simulink model "stateflow_incrementsaction"  (R2015b)
settings: Solver=VariableStepAuto  StartTime=0.0  StopTime=10.0  RelTol=1e-3
settings Model: Creator=amyyang  LastModifiedBy=amyyang

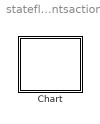
== system stateflow_incrementsaction ==
  Chart : Stateflow chart  TreatAsAtomicUnit=on

== stateflow chart stateflow_incrementsaction/Chart ==
  note: 条件语句里面必须是返回布尔量
  note: 条件语句里面必须是返回布尔量
  note: 禁止这样写
  note: 在索引里建议不要使用表达式
  note: 禁止这样写
  note: 不要使用非布尔量作为条件
  (junction 1) -> (junction 2) : {
      |  k++;
      | a = out[k];
      | }
  (junction 21) -> (junction 20) : {
      |  k = k + 5;
      | a = out[k];
      | }
  (junction 27) -> (junction 28) : [ indata == 1]
  (default) -> (junction 4) [order 1] : {
      |  u16_ver2++;
      | }
  (junction 4) -> (junction 6) : [u16_ver1 == u16_ver2]
  (junction 28) -> (junction 29) : [ indataBoolean ]
  (junction 11) -> (junction 10) : {
      | a = out[k++];
      | }
  (junction 22) -> (junction 24) : {
      |
      | a = out[k + 5];
      | }
  (default) -> (junction 13) [order 2]
  (junction 29) -> (junction 32) : [ indataUint8]
  (junction 13) -> (junction 14) : [u16_ver1 == (u16_ver2++)]
